simulink model "encoder_1"  (Simulink 6.0)
settings: Solver=FixedStepDiscrete  SolverMode=SingleTasking  StartTime=0.0  StopTime=1  FixedStep=1/8000  MaxStep=1/8000  RelTol=1e-3
values from neighbouring files (symbols this model uses):
  A = sqrt(a(k)^2+b(k)^2)    [AbyS.m]    (also in recons_residual.m = sqrt(a_np.^2+b_np.^2))
undefined symbols (not defined in the file or in its folder): error_weighting, magnitude
libraries: simulink x10, dspmtrx3 x6, dspbuff3 x5, dspsnks4 x5, dsplp x3, dsparch4 x3, dspindex x2, dspquant2 x2, dspobslib x2, dspsigops x1, dspsolvers x1, dspstat3 x1
settings Model: LastModifiedBy=Paulo

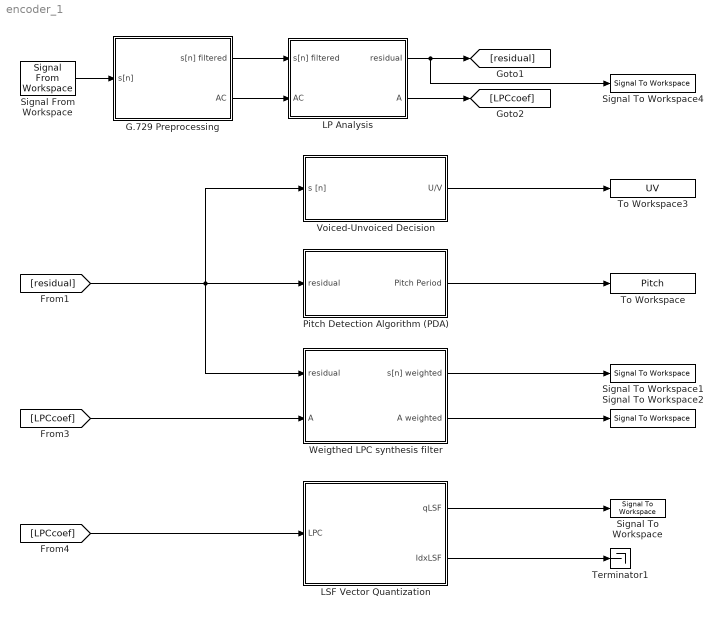
== system encoder_1 ==
  G.729 Preprocessing : Subsystem
  LP Analysis : Subsystem
  LSF Vector Quantization : Subsystem
  Pitch Detection Algorithm (PDA) : Subsystem
  Signal From Workspace : dspsrcs4/Signal From Workspace  X=speech  Ts=1/8000  nsamps=80  OutputAfterFinalValue=Setting to zero
  Signal To Workspace : dspsnks4/Signal To Workspace  VariableName=LSFs  FrameMode=Concatenate frames (2-D array)
      settings: FixptAsFi=off
  Signal To Workspace1 : dspsnks4/Signal To Workspace  VariableName=SignalWeighted  FrameMode=Concatenate frames (2-D array)
      settings: FixptAsFi=off
  Signal To Workspace2 : dspsnks4/Signal To Workspace  VariableName=LPCWeighted  FrameMode=Concatenate frames (2-D array)
      settings: FixptAsFi=off
  Signal To Workspace4 : dspsnks4/Signal To Workspace  VariableName=residual  FrameMode=Concatenate frames (2-D array)
      settings: FixptAsFi=off
  Terminator1 : Terminator
  To Workspace : ToWorkspace  VariableName=Pitch  SampleTime=-1  SaveFormat=Array
  To Workspace3 : ToWorkspace  VariableName=UV  SampleTime=-1  SaveFormat=Array
  Voiced-Unvoiced Decision : Subsystem
  Weigthed LPC synthesis filter : Subsystem
  wires:
  LP Analysis/2(A) -> [LPCcoef]
  Pitch Detection Algorithm (PDA)/1(Pitch Period) -> To Workspace/1
  G.729 Preprocessing/2(AC) -> LP Analysis/2(AC)
  G.729 Preprocessing/1("s[n] filtered ") -> LP Analysis/1(s[n] filtered)
  LP Analysis/1(residual) -> [residual], Signal To Workspace4/1
  Weigthed LPC synthesis filter/1(s[n] weighted) -> Signal To Workspace1/1
  Weigthed LPC synthesis filter/2(A weighted) -> Signal To Workspace2/1
  Voiced-Unvoiced Decision/1(U/V) -> To Workspace3/1
  Signal From Workspace/1 -> G.729 Preprocessing/1(s[n])
  [residual] -> Pitch Detection Algorithm (PDA)/1(residual), Weigthed LPC synthesis filter/1(residual), Voiced-Unvoiced Decision/1(s [n])
  [LPCcoef] -> Weigthed LPC synthesis filter/2(A)
  LSF Vector Quantization/1(qLSF) -> Signal To Workspace/1
  [LPCcoef] -> LSF Vector Quantization/1(LPC)
  LSF Vector Quantization/2(IdxLSF) -> Terminator1/1

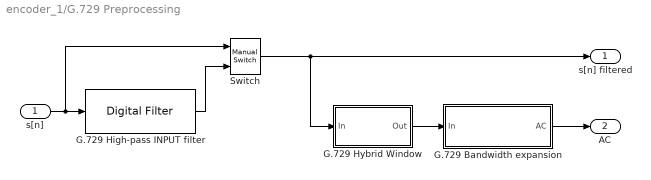
== system encoder_1/G.729 Preprocessing ==
  s[n] : Inport  Port=1  LatchInput=off
  G.729 Bandwidth expansion : Subsystem
  G.729 High-pass INPUT filter : dsparch4/Digital Filter  DialogController=dspDDGCreate  DialogControllerArgs=DataTag1  TypePopup=IIR (poles & zeros)  IIRFiltStruct=Direct form II transposed  AllPoleFiltStruct=Direct form  FIRFiltStruct=Direct form  CoeffSource=Specify via dialog  NumCoeffs=[0.4636718 -0.92724705 0.4636718]  DenCoeffs=[1 1.19059465 0.9114024]  BiQuadCoeffs=[1 0.3 0.4 1 0.1 0.2]  LatticeCoeffs=[0.2 0.4]  denIgnore=on  FiltPerSampPopup=One filter per frame  IC=0  ICnum=0  ICden=0  roundingMode=Floor  overflowMode=off  ScaleValues=1  scaleValueFracLength=14  stageInFracLength=15  stageOutFracLength=15
  G.729 Hybrid Window : Subsystem
  Switch : simulink/Signal Routing/Manual Switch  sw=1  action=0
  "s[n] filtered " : Outport
  AC : Outport  Port=2
  wires:
  G.729 Bandwidth expansion/1(AC) -> AC/1
  G.729 Hybrid Window/1(Out) -> G.729 Bandwidth expansion/1(In)
  s[n]/1 -> G.729 High-pass INPUT filter/1, Switch/1
  Switch/1 -> G.729 Hybrid Window/1(In), "s[n] filtered "/1
  G.729 High-pass INPUT filter/1 -> Switch/2

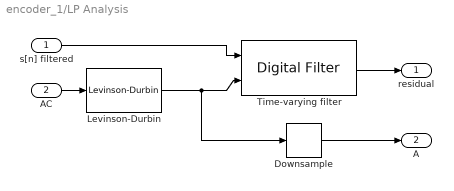
== system encoder_1/LP Analysis ==
  s[n] filtered : Inport  Port=1  LatchInput=off
  AC : Inport  Port=2  LatchInput=off
  Downsample : dspsigops/Downsample  N=2  phase=0  ic=0  smode=Allow multirate  fmode=Maintain input frame size
  Levinson-Durbin : dspsolvers/Levinson-Durbin  DialogController=dspDDGCreate  DialogControllerArgs=DataTag3  coeffOutFcn=A  outP=off  zeroInpHandling=on  firstCoeffMode=Binary point scaling  firstCoeffWordLength=16  firstCoeffFracLength=15  secondCoeffMode=Binary point scaling  secondCoeffWordLength=16  secondCoeffFracLength=15  accumMode=Binary point scaling  accumWordLength=32  accumFracLength=30  prodOutputMode=Binary point scaling  prodOutputWordLength=32  prodOutputFracLength=30  roundingMode=Floor  overflowMode=off
      settings: allowOverrides=off
  Time-varying filter : dsparch4/Digital Filter  DialogController=dspDDGCreate  DialogControllerArgs=DataTag4  TypePopup=FIR (all zeros)  IIRFiltStruct=Direct form II transposed  AllPoleFiltStruct=Direct form  FIRFiltStruct=Direct form  CoeffSource=Input port(s)  NumCoeffs=[0.4636718 -0.92724705 0.4636718]  DenCoeffs=[1 1.19059465 0.9114024]  BiQuadCoeffs=[1 0.3 0.4 1 0.1 0.2]  LatticeCoeffs=[0.2 0.4]  denIgnore=on  FiltPerSampPopup=One filter per frame  IC=0  ICnum=0  ICden=0  roundingMode=Floor  overflowMode=off  ScaleValues=1  scaleValueFracLength=14  stageInFracLength=15  stageOutFracLength=15
  residual : Outport
  A : Outport  Port=2
  wires:
  Levinson-Durbin/1 -> Time-varying filter/2, Downsample/1
  s[n] filtered/1 -> Time-varying filter/1
  Time-varying filter/1 -> residual/1
  AC/1 -> Levinson-Durbin/1
  Downsample/1 -> A/1

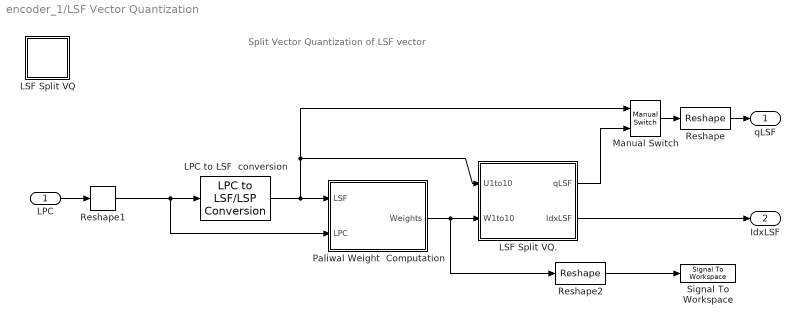
== system encoder_1/LSF Vector Quantization ==
  note: Split Vector Quantization of LSF vector
  LPC : Inport  Port=1  LatchInput=off
  LPC to LSF  conversion : dsplp/LPC to LSF//LSP Conversion  output=LSF in range (0 pi)  NSteps=64  NBisects=4  RootStatus=off  correction=off  lastLSP=off  error=Ignore
  LSF Split VQ : Subsystem  mask(DocBlock){ECoderFlag=, DocumentType=Text}
      mask prompts: ECoderFlag "RTW Embedded Coder Flag"; DocumentType "Document Type"
      mask help: Use this block to save long descriptive text with the model. Double-clicking the block will open an editor.
      settings: CopyFcn=docblock('breaklink',gcb);  DeleteFcn=docblock('close_document',gcb);  PreSaveFcn=docblock('save_document',gcb);  OpenFcn=docblock('edit_document',gcb);
      mask StyleString: edit,popup(Text|RTF|HTML)
      mask Display:
      | plot([.8 0 0 1 1 .8 .8 1],[1 1 0 0 .8 1 .8 .8]);
      | text(.5,.5,'DOC','horizontalalignment','center');
  LSF Split VQ. : Subsystem
  Manual Switch : simulink/Signal Routing/Manual Switch  sw=1  action=0
  Paliwal Weight  Computation : Subsystem
  Reshape : simulink/Math Operations/Reshape  OutputDimensionality=1-D array  OutputDimensions=[10,1]
  Reshape1 : simulink/Math Operations/Reshape  OutputDimensionality=Column vector  OutputDimensions=[1,1]
  Reshape2 : simulink/Math Operations/Reshape  OutputDimensionality=1-D array  OutputDimensions=[10,1]
  Signal To Workspace : dspsnks4/Signal To Workspace  VariableName=Weights  FrameMode=Concatenate frames (2-D array)
      settings: FixptAsFi=off
  qLSF : Outport
  IdxLSF : Outport  Port=2
  wires:
  LPC/1 -> Reshape1/1
  Paliwal Weight  Computation/1(Weights) -> LSF Split VQ./2(W1to10), Reshape2/1
  Reshape1/1 -> LPC to LSF  conversion/1, Paliwal Weight  Computation/2(LPC)
  LPC to LSF  conversion/1 -> Paliwal Weight  Computation/1(LSF), LSF Split VQ./1(U1to10), Manual Switch/1
  LSF Split VQ./1(qLSF) -> Manual Switch/2
  Manual Switch/1 -> Reshape/1
  LSF Split VQ./2(IdxLSF) -> IdxLSF/1
  Reshape/1 -> qLSF/1
  Reshape2/1 -> Signal To Workspace/1

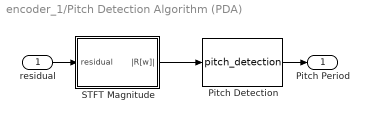
== system encoder_1/Pitch Detection Algorithm (PDA) ==
  residual : Inport  Port=1  LatchInput=off
  Pitch Detection : MATLABFcn  MATLABFcn=pitch_detection
  STFT Magnitude : Subsystem
  Pitch Period : Outport
  wires:
  STFT Magnitude/1(|R[w]|) -> Pitch Detection/1
  Pitch Detection/1 -> Pitch Period/1
  residual/1 -> STFT Magnitude/1(residual)

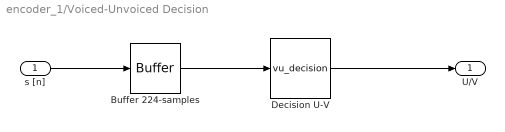
== system encoder_1/Voiced-Unvoiced Decision ==
  s [n] : Inport  Port=1  LatchInput=off
  Buffer 224-samples : dspbuff3/Buffer  N=224  V=64  ic=0
  Decision U-V : MATLABFcn  MATLABFcn=vu_decision  Output1D=off
  U/V : Outport
  wires:
  Decision U-V/1 -> U/V/1
  Buffer 224-samples/1 -> Decision U-V/1
  s [n]/1 -> Buffer 224-samples/1

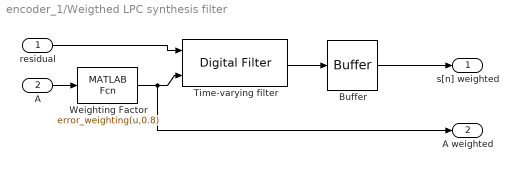
== system encoder_1/Weigthed LPC synthesis filter ==
  residual : Inport  Port=1  LatchInput=off
  A : Inport  Port=2  LatchInput=off
  Buffer : dspbuff3/Buffer  N=160  V=0  ic=0
  Time-varying filter : dsparch4/Digital Filter  DialogController=dspDDGCreate  DialogControllerArgs=DataTag7  TypePopup=IIR (all poles)  IIRFiltStruct=Direct form II transposed  AllPoleFiltStruct=Direct form  FIRFiltStruct=Direct form  CoeffSource=Input port(s)  NumCoeffs=[0.4636718 -0.92724705 0.4636718]  DenCoeffs=[1 1.19059465 0.9114024]  BiQuadCoeffs=[1 0.3 0.4 1 0.1 0.2]  LatticeCoeffs=[0.2 0.4]  denIgnore=on  FiltPerSampPopup=One filter per frame  IC=0  ICnum=0  ICden=0  roundingMode=Floor  overflowMode=off  ScaleValues=1  scaleValueFracLength=14  stageInFracLength=15  stageOutFracLength=15
  Weighting Factor : MATLABFcn  MATLABFcn=error_weighting(u,0.8)
  s[n] weighted : Outport
  A weighted : Outport  Port=2
  wires:
  Weighting Factor/1 -> Time-varying filter/2, A weighted/1
  residual/1 -> Time-varying filter/1
  Time-varying filter/1 -> Buffer/1
  A/1 -> Weighting Factor/1
  Buffer/1 -> s[n] weighted/1

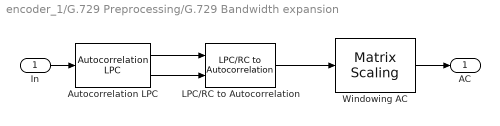
== system encoder_1/G.729 Preprocessing/G.729 Bandwidth expansion ==
  In : Inport  Port=1  LatchInput=off
  Autocorrelation LPC : dsplp/Autocorrelation LPC  lpcCoeffOutFcn=A  lpcOutP=on  inherit_prediction_order=off  order=10
  LPC/RC to Autocorrelation : dsplp/LPC//RC to Autocorrelation  conversion=LPC to autocorrelation  perr_spec=Via input port  error=Replace it with 1
  Windowing AC : dspmtrx3/Matrix Scaling  DialogController=dspDDGCreate  DialogControllerArgs=DataTag0  mode=Scale rows (D*A)  D_Source=Dialog parameter  D_VectFromMask=bandwidth_expansion  roundingMode=Floor  overflowMode=off
  AC : Outport
  wires:
  Autocorrelation LPC/1 -> LPC/RC to Autocorrelation/1
  Windowing AC/1 -> AC/1
  Autocorrelation LPC/2 -> LPC/RC to Autocorrelation/2
  LPC/RC to Autocorrelation/1 -> Windowing AC/1
  In/1 -> Autocorrelation LPC/1

== system encoder_1/G.729 Preprocessing/G.729 Hybrid Window ==
  note: El buffer agrega
      | un retardo
      | de 40 muestras
  In : Inport  Port=1  LatchInput=off
  Buffer 240-samples : dspbuff3/Buffer  N=240  V=160  ic=0
  Windowing : dspmtrx3/Matrix Scaling  DialogController=dspDDGCreate  DialogControllerArgs=DataTag2  mode=Scale rows (D*A)  D_Source=Dialog parameter  D_VectFromMask=hybrid_window  roundingMode=Floor  overflowMode=off
  Out : Outport
  wires:
  Buffer 240-samples/1 -> Windowing/1
  In/1 -> Buffer 240-samples/1
  Windowing/1 -> Out/1

== system encoder_1/LSF Vector Quantization/LSF Split VQ ==
  EmptySubsystem : Subsystem

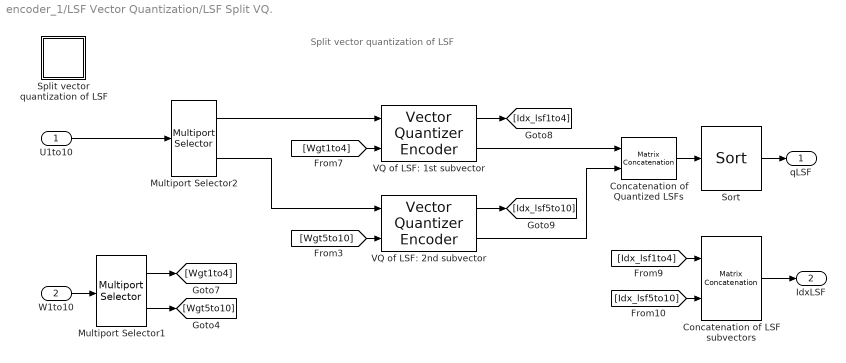
== system encoder_1/LSF Vector Quantization/LSF Split VQ. ==
  note: Split vector quantization of LSF
  U1to10 : Inport  Port=1  LatchInput=off
  W1to10 : Inport  Port=2  LatchInput=off
  Concatenation of LSF subvectors : simulink/Math Operations/Matrix Concatenation  numInports=2  catMethod=Horizontal
  Concatenation of Quantized LSFs : simulink/Math Operations/Matrix Concatenation  numInports=2  catMethod=Vertical
  Multiport Selector1 : dspindex/Multiport Selector  rowsOrCols=Rows  idxCellArray={1:4,5:10}  idxErrMode=Clip Index
  Multiport Selector2 : dspindex/Multiport Selector  rowsOrCols=Rows  idxCellArray={1:4,5:10}  idxErrMode=Clip Index
  Sort : dspstat3/Sort  DialogController=dspDDGCreate  DialogControllerArgs=DataTag5  otype=Value  dir=Ascending  sortAlg=Quick sort  roundingMode=Floor  overflowMode=off
  Split vector quantization of LSF : Subsystem  mask(DocBlock){ECoderFlag=, DocumentType=Text}
      mask prompts: ECoderFlag "RTW Embedded Coder Flag"; DocumentType "Document Type"
      mask help: Use this block to save long descriptive text with the model. Double-clicking the block will open an editor.
      settings: CopyFcn=docblock('breaklink',gcb);  DeleteFcn=docblock('close_document',gcb);  PreSaveFcn=docblock('save_document',gcb);  OpenFcn=docblock('edit_document',gcb);
      mask StyleString: edit,popup(Text|RTF|HTML)
      mask Display:
      | plot([.8 0 0 1 1 .8 .8 1],[1 1 0 0 .8 1 .8 .8]);
      | text(.5,.5,'DOC','horizontalalignment','center');
  VQ of LSF: 1st subvector : dspquant2/Vector Quantizer Encoder  CBsource=Specify via dialog  codebook=CB_LSF_1to4  distMeasure=Weighted squared error  wgtSrc=Input port  weights=[1 1 1]  tieBreakRule=Choose the lower index  outQU=on  outQError=off  idtype=int32  roundingMode=Floor  overflowMode=off
  VQ of LSF: 2nd subvector : dspquant2/Vector Quantizer Encoder  CBsource=Specify via dialog  codebook=CB_LSF_5to10  distMeasure=Weighted squared error  wgtSrc=Input port  weights=[1 1 1]  tieBreakRule=Choose the lower index  outQU=on  outQError=off  idtype=int32  roundingMode=Floor  overflowMode=off
  qLSF : Outport
  IdxLSF : Outport  Port=2
  wires:
  VQ of LSF: 1st subvector/2 -> Concatenation of Quantized LSFs/1
  VQ of LSF: 1st subvector/1 -> [Idx_lsf1to4]
  Multiport Selector2/2 -> VQ of LSF: 2nd subvector/1
  Multiport Selector1/2 -> [Wgt5to10]
  VQ of LSF: 2nd subvector/1 -> [Idx_lsf5to10]
  VQ of LSF: 2nd subvector/2 -> Concatenation of Quantized LSFs/2
  Concatenation of Quantized LSFs/1 -> Sort/1
  [Wgt5to10] -> VQ of LSF: 2nd subvector/2
  Multiport Selector1/1 -> [Wgt1to4]
  [Wgt1to4] -> VQ of LSF: 1st subvector/2
  [Idx_lsf1to4] -> Concatenation of LSF subvectors/1
  [Idx_lsf5to10] -> Concatenation of LSF subvectors/2
  W1to10/1 -> Multiport Selector1/1
  U1to10/1 -> Multiport Selector2/1
  Sort/1 -> qLSF/1
  Concatenation of LSF subvectors/1 -> IdxLSF/1
  Multiport Selector2/1 -> VQ of LSF: 1st subvector/1

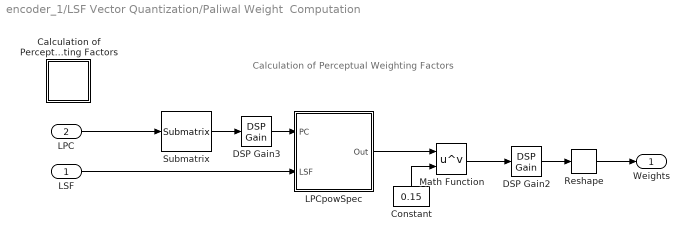
== system encoder_1/LSF Vector Quantization/Paliwal Weight  Computation ==
  note: Calculation of Perceptual Weighting Factors
  LSF : Inport  Port=1  LatchInput=off
  LPC : Inport  Port=2  LatchInput=off
  Calculation of Perceptual  Weighting Factors : Subsystem  mask(DocBlock){ECoderFlag=, DocumentType=Text}
      mask prompts: ECoderFlag "RTW Embedded Coder Flag"; DocumentType "Document Type"
      mask help: Use this block to save long descriptive text with the model. Double-clicking the block will open an editor.
      settings: CopyFcn=docblock('breaklink',gcb);  DeleteFcn=docblock('close_document',gcb);  PreSaveFcn=docblock('save_document',gcb);  OpenFcn=docblock('edit_document',gcb);
      mask StyleString: edit,popup(Text|RTF|HTML)
      mask Display:
      | plot([.8 0 0 1 1 .8 .8 1],[1 1 0 0 .8 1 .8 .8]);
      | text(.5,.5,'DOC','horizontalalignment','center');
  Constant : Constant  Orientation=up  Value=0.15  VectorParams1D=off  SampleTime=1/50
  DSP Gain2 : dspobslib/DSP Gain  gainValue=[ones(1,8) 0.8 0.4]  roundingMode=Floor  overflowMode=off
  DSP Gain3 : dspobslib/DSP Gain  gainValue=-1  roundingMode=Floor  overflowMode=off
  LPCpowSpec : Subsystem
  Math Function : Math  Operator=pow  SaturateOnIntegerOverflow=on
  Reshape : simulink/Math Operations/Reshape  OutputDimensionality=Column vector  OutputDimensions=[1,1]
  Submatrix : dspmtrx3/Submatrix  RowSpan=Range of rows  RowStartMode=Index  RowStartIndex=2  RowEndMode=Last  RowEndIndex=1  ColSpan=All columns  ColStartMode=First  ColStartIndex=1  ColEndMode=Last  ColEndIndex=1
  Weights : Outport
  wires:
  LPCpowSpec/1(Out) -> Math Function/1
  Constant/1 -> Math Function/2
  Math Function/1 -> DSP Gain2/1
  DSP Gain2/1 -> Reshape/1
  LSF/1 -> LPCpowSpec/2(LSF)
  Reshape/1 -> Weights/1
  Submatrix/1 -> DSP Gain3/1
  LPC/1 -> Submatrix/1
  DSP Gain3/1 -> LPCpowSpec/1(PC)

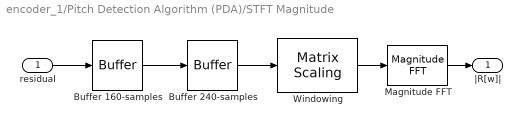
== system encoder_1/Pitch Detection Algorithm (PDA)/STFT Magnitude ==
  residual : Inport  Port=1  LatchInput=off
  Buffer 160-samples : dspbuff3/Buffer  N=160  V=0  ic=0
  Buffer 240-samples : dspbuff3/Buffer  N=240  V=80  ic=0
  Magnitude FFT : dspspect3/Magnitude FFT  mag_or_magsq=Magnitude  fftLenInherit=off  fftsize=512
  Windowing : dspmtrx3/Matrix Scaling  DialogController=dspDDGCreate  DialogControllerArgs=DataTag6  mode=Scale rows (D*A)  D_Source=Dialog parameter  D_VectFromMask=hamming(240)  roundingMode=Floor  overflowMode=off
  |R[w]| : Outport
  wires:
  Buffer 240-samples/1 -> Windowing/1
  Windowing/1 -> Magnitude FFT/1
  residual/1 -> Buffer 160-samples/1
  Magnitude FFT/1 -> |R[w]|/1
  Buffer 160-samples/1 -> Buffer 240-samples/1

== system encoder_1/LSF Vector Quantization/LSF Split VQ/EmptySubsystem ==

== system encoder_1/LSF Vector Quantization/LSF Split VQ./Split vector quantization of LSF ==
  EmptySubsystem : Subsystem

== system encoder_1/LSF Vector Quantization/Paliwal Weight  Computation/Calculation of Perceptual  Weighting Factors ==
  EmptySubsystem : Subsystem

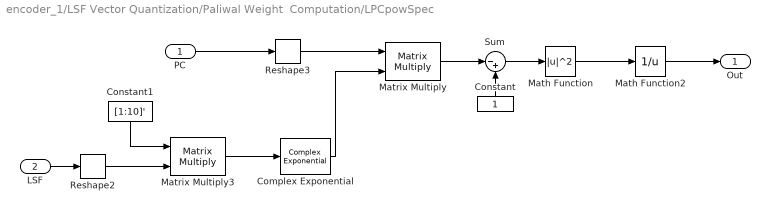
== system encoder_1/LSF Vector Quantization/Paliwal Weight  Computation/LPCpowSpec ==
  PC : Inport  Port=1  LatchInput=off
  LSF : Inport  Port=2  LatchInput=off
  Complex Exponential : dspmathops/Complex Exponential
  Constant : Constant  Orientation=up  VectorParams1D=off  SampleTime=1/50
  Constant1 : Constant  Orientation=down  Value=[1:10]'  VectorParams1D=off  SampleTime=1/50
  Math Function : Math  Operator=magnitude^2  SaturateOnIntegerOverflow=on
  Math Function2 : Math  Operator=reciprocal  SaturateOnIntegerOverflow=on
  Matrix Multiply : dspmtrx3/Matrix Multiply  numInputPorts=2  OptimizationLevel=None
  Matrix Multiply3 : dspmtrx3/Matrix Multiply  numInputPorts=2  OptimizationLevel=None
  Reshape2 : simulink/Math Operations/Reshape  OutputDimensionality=Row vector  OutputDimensions=[1,1]
  Reshape3 : simulink/Math Operations/Reshape  OutputDimensionality=Row vector  OutputDimensions=[1,1]
  Sum : Sum  Inputs=|-+  SaturateOnIntegerOverflow=on
  Out : Outport
  wires:
  Math Function2/1 -> Out/1
  Matrix Multiply/1 -> Sum/1
  PC/1 -> Reshape3/1
  Complex Exponential/1 -> Matrix Multiply/2
  Math Function/1 -> Math Function2/1
  Sum/1 -> Math Function/1
  Constant/1 -> Sum/2
  Reshape3/1 -> Matrix Multiply/1
  LSF/1 -> Reshape2/1
  Reshape2/1 -> Matrix Multiply3/2
  Constant1/1 -> Matrix Multiply3/1
  Matrix Multiply3/1 -> Complex Exponential/1

== system encoder_1/LSF Vector Quantization/LSF Split VQ./Split vector quantization of LSF/EmptySubsystem ==

== system encoder_1/LSF Vector Quantization/Paliwal Weight  Computation/Calculation of Perceptual  Weighting Factors/EmptySubsystem ==
